simulink model "Houghline_real"  (R2016a)
settings: Solver=VariableStepAuto  StartTime=0.0  StopTime=inf  RelTol=1e-3
undefined symbols (not defined in the file): gray, strel
libraries: visionanalysis x5, visiontransforms x3, visionmorphops x2, visiontextngfix x2, dspvision x1, visionstatistics x1, visionconversions x1
settings Model: Creator=Yewly  LastModifiedBy=Yewly
settings GRTTargetCC: GeneratePreprocessorConditionals=Use local settings

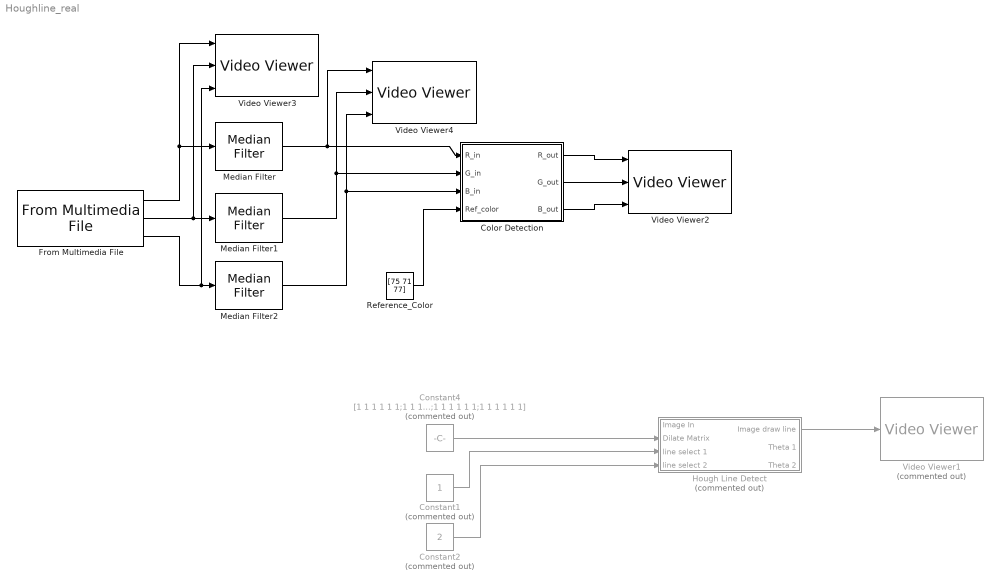
== system Houghline_real ==
  Color Detection : Subsystem
  Constant1 : Constant  Commented=on  OutDataTypeStr=double
  Constant2 : Constant  Commented=on  Value=2  OutDataTypeStr=double
  Constant4 : Constant  Commented=on  Value=[1 1 1 1 1 1;1 1 1 1 1 1;1 1 1 1 1 1;1 1 1 1 1 1;1 1 1 1 1 1;1 1 1 1 1 1]  OutDataTypeStr=boolean
  From Multimedia File : dspvision/From Multimedia File  inputFilename=lane2.mp4  loop=on  numPlays=inf  outputStreams=Video only  videoDataType=single  audioDataType=int16  inheritSampleTime=on  userDefinedSampleTime=1/30  noAudioOutput=off  isIntensityVideo=off  fourcc=RGB  colorVideoFormat=Separate color signals  outputEOF=off  dataOrg=Column-major  audioFrameSize=1024  computeAudioFrameSize=off  outSamplingMode=Sample based
  "Hough Line Detect " : Subsystem  Commented=on
  Median Filter : visionanalysis/Median Filter  nghbood=[11 11]  outSize=Same as input port I  padType=Symmetric  padSrc=Specify via dialog  padVal=0  roundingMode=Floor  overflowMode=off
  Median Filter1 : visionanalysis/Median Filter  nghbood=[11 11]  outSize=Same as input port I  padType=Symmetric  padSrc=Specify via dialog  padVal=0  roundingMode=Floor  overflowMode=off
  Median Filter2 : visionanalysis/Median Filter  nghbood=[11 11]  outSize=Same as input port I  padType=Symmetric  padSrc=Specify via dialog  padVal=0  roundingMode=Floor  overflowMode=off
  Reference_Color : Constant  Value=[75 71 77]  OutDataTypeStr=uint8
  Video Viewer1 : VideoViewer  Commented=on  colormapValue=gray(256)  FigPos=[596.2 615.6 714.4 445.6]
  Video Viewer2 : VideoViewer  imagePorts=separate color signals  colormapValue=gray(256)  FigPos=[459.4 708.4 714.4 445.6]
  Video Viewer3 : VideoViewer  imagePorts=separate color signals  colormapValue=gray(256)  FigPos=[752.2 654.8 714.4 445.6]
  Video Viewer4 : VideoViewer  imagePorts=separate color signals  colormapValue=gray(256)  FigPos=[113.8 832.4 714.4 445.6]
  wires:
  Constant4/1 -> "Hough Line Detect "/2("Dilate Matrix ")
  "Hough Line Detect "/1("Image draw line ") -> Video Viewer1/1
  Constant1/1 -> "Hough Line Detect "/3(line select 1)
  Constant2/1 -> "Hough Line Detect "/4(line select 2)
  From Multimedia File/1 -> Video Viewer3/1, Median Filter/1
  From Multimedia File/2 -> Video Viewer3/2, Median Filter1/1
  From Multimedia File/3 -> Video Viewer3/3, Median Filter2/1
  Median Filter/1 -> Color Detection/1(R_in), Video Viewer4/1
  Median Filter1/1 -> Color Detection/2(G_in), Video Viewer4/2
  Median Filter2/1 -> Color Detection/3(B_in), Video Viewer4/3
  Reference_Color/1 -> Color Detection/4(Ref_color)
  Color Detection/1(R_out) -> Video Viewer2/1
  Color Detection/2(G_out) -> Video Viewer2/2
  Color Detection/3(B_out) -> Video Viewer2/3

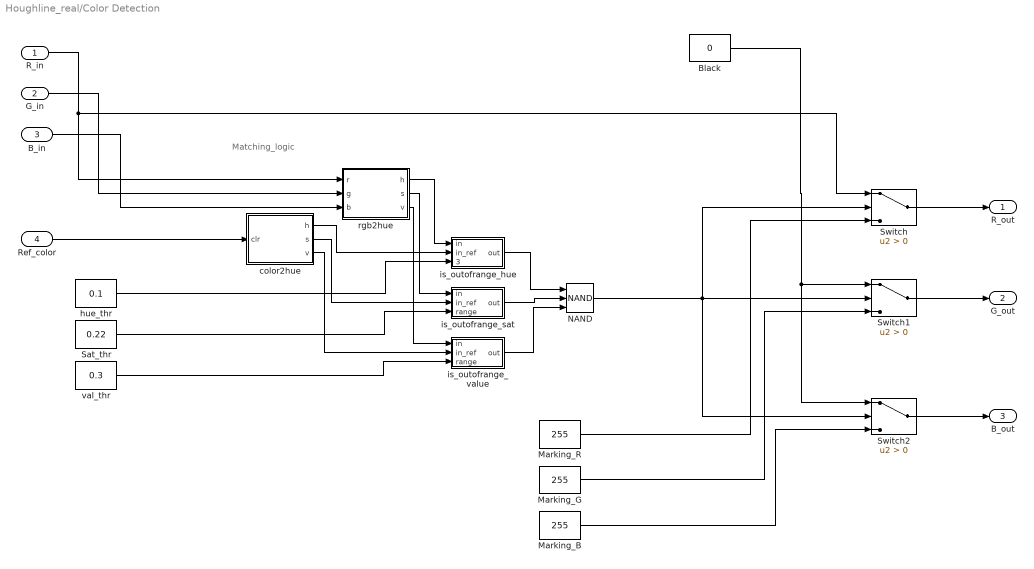
== system Houghline_real/Color Detection ==
  note: Matching_logic
  R_in : Inport
  G_in : Inport  Port=2
  B_in : Inport  Port=3
  Ref_color : Inport  Port=4
  "Black " : Constant  Value=0
  Marking_B : Constant  Value=255
  Marking_G : Constant  Value=255
  Marking_R : Constant  Value=255
  NAND : Logic  Operator=NAND  Inputs=3  IconShape=distinctive  AllPortsSameDT=off  OutDataTypeStr=boolean
  Sat_thr : Constant  Value=0.22
  Switch : Switch  Criteria=u2 > Threshold  OutDataTypeStr=uint8
  Switch1 : Switch  Criteria=u2 > Threshold  OutDataTypeStr=uint8
  Switch2 : Switch  Criteria=u2 > Threshold  OutDataTypeStr=uint8
  color2hue : MATLAB Function  TreatAsAtomicUnit=on
  hue_thr : Constant  Value=0.1
  is_outofrange_hue : Subsystem
  "is_outofrange_sat " : Subsystem
  is_outofrange_value : Subsystem
  rgb2hue : MATLAB Function  TreatAsAtomicUnit=on
  val_thr : Constant  Value=0.3
  R_out : Outport
  G_out : Outport  Port=2
  B_out : Outport  Port=3
  wires:
  NAND/1 -> Switch2/2, Switch1/2, Switch/2
  hue_thr/1 -> is_outofrange_hue/3("threshold ")
  is_outofrange_value/1(out) -> NAND/3
  is_outofrange_hue/1(out) -> NAND/1
  Sat_thr/1 -> "is_outofrange_sat "/3("range ")
  val_thr/1 -> is_outofrange_value/3("range ")
  rgb2hue/3(v) -> is_outofrange_value/1(in)
  color2hue/3(v) -> is_outofrange_value/2(in_ref)
  color2hue/1(h) -> is_outofrange_hue/2(in_ref)
  rgb2hue/1(h) -> is_outofrange_hue/1(in)
  Ref_color/1 -> color2hue/1(clr)
  "is_outofrange_sat "/1(out) -> NAND/2
  color2hue/2(s) -> "is_outofrange_sat "/2(in_ref)
  G_in/1 -> rgb2hue/2(g)
  rgb2hue/2(s) -> "is_outofrange_sat "/1(in)
  B_in/1 -> rgb2hue/3(b)
  R_in/1 -> Switch/1, rgb2hue/1(r)
  Marking_R/1 -> Switch/3
  Switch/1 -> R_out/1
  Switch1/1 -> G_out/1
  Switch2/1 -> B_out/1
  Marking_G/1 -> Switch1/3
  Marking_B/1 -> Switch2/3
  "Black "/1 -> Switch2/1, Switch1/1

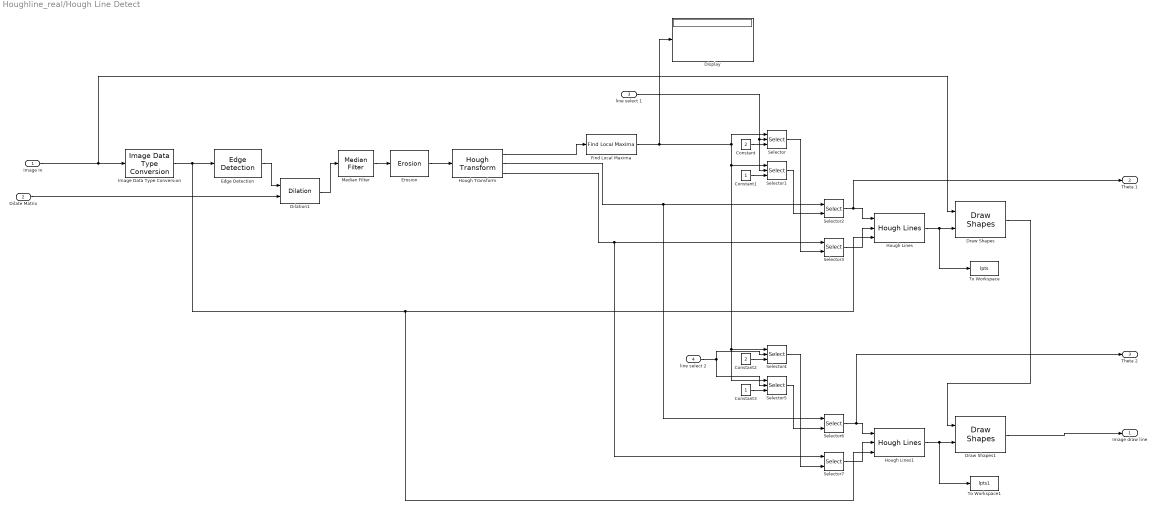
== system Houghline_real/Hough Line Detect  ==
  Image In : Inport
  "Dilate Matrix " : Inport  Port=2
  line select 1 : Inport  Port=3
  line select 2 : Inport  Port=4
  Constant : Constant  Value=2
  Constant1 : Constant
  Constant2 : Constant  Value=2
  Constant3 : Constant
  Dilation1 : visionmorphops/Dilation  nhoodsrc=Input port  strel=[1 1 1 1 1 1;1 1 1 1 1 1;1 1 1 1 1 1;1 1 1 1 1 1;1 1 1 1 1 1;1 1 1 1 1 1]
  Display : Display
  Draw Shapes : visiontextngfix/Draw Shapes  shape=Lines  fill=off  lineWidth=10  fillClrSource=Specify via dialog  display=White  intensity=200  color=255  opacity=0.6  viewport=Entire image  antialiasing=off  inType=Obsolete  imagePorts=One multidimensional signal  prodOutputMode=Binary point scaling  prodOutputWordLength=32  prodOutputFracLength=14  memoryMode=Specify word length  memoryWordLength=16  memoryFracLength=14  roundingMode=Floor  overflowMode=off
  Draw Shapes1 : visiontextngfix/Draw Shapes  shape=Lines  fill=off  lineWidth=10  fillClrSource=Specify via dialog  display=White  intensity=200  color=255  opacity=0.6  viewport=Entire image  antialiasing=off  inType=Obsolete  imagePorts=One multidimensional signal  prodOutputMode=Binary point scaling  prodOutputWordLength=32  prodOutputFracLength=14  memoryMode=Specify word length  memoryWordLength=16  memoryFracLength=14  roundingMode=Floor  overflowMode=off
  Edge Detection : visionanalysis/Edge Detection  method=Sobel  outputType=Binary image  userDefinedThreshold=off  thresholdSource=Input port  threshold=20  thresholdTuning=4  edgeThinning=on  threshold_canny=[0.25 0.60]  autoPercent=70  sigma=1  prodOutputMode=Binary point scaling  prodOutputWordLength=32  prodOutputFracLength=8  roundingMode=Floor  overflowMode=off
  Erosion : visionmorphops/Erosion  nhoodsrc=Specify via dialog  strel=strel('square',12)
  Find Local Maxima : visionstatistics/Find Local Maxima  num_peaks=5  nhood_size=[5 7]  src_thresh=Obsolete9b  src_thresh_inuse=Specify via dialog  threshold=10  inputIsHough=on  dt_peak=uint32  isOutVarDim=on  dt_count=uint32
  Hough Lines : visiontransforms/Hough Lines  sineCompMethod=Trigonometric function  thetaRes=pi/180  firstCoeffMode=Specify word length  firstCoeffWordLength=16  firstCoeffFracLength=15  prodOutputMode=Binary point scaling  prodOutputWordLength=32  prodOutputFracLength=16  roundingMode=Nearest  overflowMode=on
  Hough Lines1 : visiontransforms/Hough Lines  sineCompMethod=Trigonometric function  thetaRes=pi/180  firstCoeffMode=Specify word length  firstCoeffWordLength=16  firstCoeffFracLength=15  prodOutputMode=Binary point scaling  prodOutputWordLength=32  prodOutputFracLength=16  roundingMode=Nearest  overflowMode=on
  Hough Transform : visiontransforms/Hough Transform  theta_res=pi/360  rho_res=1  out_theta_rho=on  outdtmode=double  firstCoeffMode=Binary point scaling  firstCoeffWordLength=16  firstCoeffFracLength=14  secondCoeffMode=Binary point scaling  secondCoeffWordLength=32  secondCoeffFracLength=16  outputMode=Binary point scaling  outputWordLength=16  outputFracLength=0  accumMode=Binary point scaling  accumWordLength=32  accumFracLength=20  prodOutputMode=Binary point scaling  prodOutputWordLength=32  prodOutputFracLength=20  memoryMode=Binary point scaling  memoryWordLength=32  memoryFracLength=16  roundingMode=Nearest  overflowMode=on
  Image Data Type Conversion : visionconversions/Image Data Type Conversion  outDT=double  isSigned=on  wordLen=16  numFracBits=0
  Median Filter : visionanalysis/Median Filter  nghbood=[3 3]  outSize=Same as input port I  padType=Symmetric  padSrc=Specify via dialog  padVal=0  roundingMode=Floor  overflowMode=off
  Selector : Selector  NumberOfDimensions=2  InputPortWidth=2  IndexOptions=Index vector (port),Index vector (port)  Indices=1,1  OutputSizes=1,1
  Selector1 : Selector  NumberOfDimensions=2  InputPortWidth=2  IndexOptions=Starting index (port),Index vector (port)  Indices=1,1  OutputSizes=1,1
  Selector{2..3,6..7} (4 alike) : Selector  NumberOfDimensions=2  InputPortWidth=3  IndexOptions=Select all,Index vector (port)  Indices=[1 3],1  OutputSizes=1,1
  Selector4 : Selector  NumberOfDimensions=2  InputPortWidth=2  IndexOptions=Index vector (port),Index vector (port)  Indices=2,1  OutputSizes=1,1
  Selector5 : Selector  NumberOfDimensions=2  InputPortWidth=2  IndexOptions=Index vector (port),Index vector (port)  Indices=2,1  OutputSizes=1,1
  To Workspace : ToWorkspace  VariableName=lpts  SampleTime=-1
  To Workspace1 : ToWorkspace  VariableName=lpts1  SampleTime=-1
  "Image draw line " : Outport
  Theta 1 : Outport  Port=2
  Theta 2 : Outport  Port=3
  wires:
  Selector5/1 -> Selector6/2
  Draw Shapes1/1 -> "Image draw line "/1
  Constant1/1 -> Selector1/3
  Constant3/1 -> Selector5/3
  Selector3/1 -> Hough Lines/2
  Hough Transform/3 -> Selector7/1, Selector3/1
  Selector4/1 -> Selector7/2
  Hough Lines/1 -> To Workspace/1, Draw Shapes/2
  Hough Transform/1 -> Find Local Maxima/1
  Edge Detection/1 -> Dilation1/1
  Selector7/1 -> Hough Lines1/2
  Hough Lines1/1 -> To Workspace1/1, Draw Shapes1/2
  Selector1/1 -> Selector2/2
  Constant2/1 -> Selector4/3
  Image In/1 -> Image Data Type Conversion/1, Draw Shapes/1
  Hough Transform/2 -> Selector6/1, Selector2/1
  Dilation1/1 -> Median Filter/1
  Selector/1 -> Selector3/2
  Erosion/1 -> Hough Transform/1
  Draw Shapes/1 -> Draw Shapes1/1
  Median Filter/1 -> Erosion/1
  "Dilate Matrix "/1 -> Dilation1/2
  Selector2/1 -> Theta 1/1, Hough Lines/1
  Selector6/1 -> Theta 2/1, Hough Lines1/1
  line select 1/1 -> Selector1/2, Selector/2
  Constant/1 -> Selector/3
  line select 2/1 -> Selector5/2, Selector4/2
  Image Data Type Conversion/1 -> Hough Lines1/3, Hough Lines/3, Edge Detection/1
  Find Local Maxima/1 -> Display/1, Selector5/1, Selector4/1, Selector1/1, Selector/1

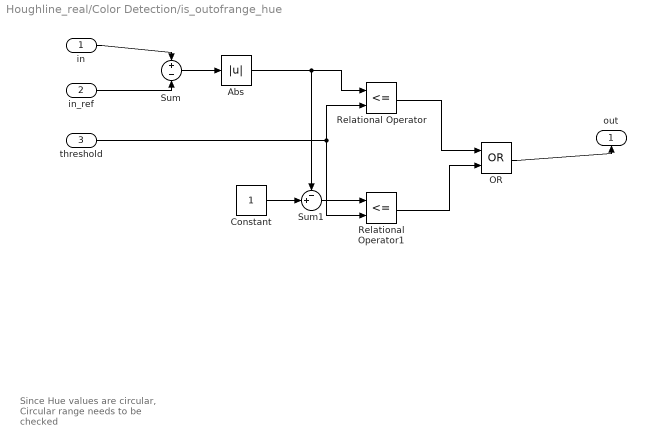
== system Houghline_real/Color Detection/is_outofrange_hue ==
  note: Since Hue values are circular, Circular range needs to be checked
  in : Inport
  in_ref : Inport  Port=2
  "threshold " : Inport  Port=3
  Abs : Abs
  Constant : Constant
  "OR " : Logic  Operator=OR  AllPortsSameDT=off  OutDataTypeStr=boolean
  Relational Operator : RelationalOperator  Operator=<=  OutDataTypeStr=boolean
  Relational Operator1 : RelationalOperator  Operator=<=  OutDataTypeStr=boolean
  Sum : Sum  Inputs=+|-
  Sum1 : Sum  Inputs=-+|
  out : Outport
  wires:
  in/1 -> Sum/1
  in_ref/1 -> Sum/2
  Sum/1 -> Abs/1
  Abs/1 -> Sum1/1, Relational Operator/1
  "threshold "/1 -> Relational Operator1/2, Relational Operator/2
  Constant/1 -> Sum1/2
  Sum1/1 -> Relational Operator1/1
  Relational Operator/1 -> "OR "/1
  Relational Operator1/1 -> "OR "/2
  "OR "/1 -> out/1

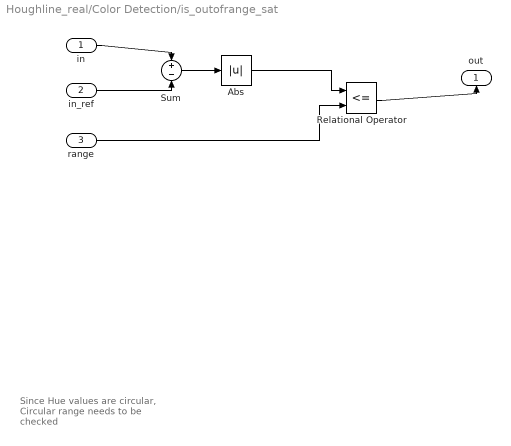
== system Houghline_real/Color Detection/is_outofrange_sat  ==
  note: Since Hue values are circular, Circular range needs to be checked
  in : Inport
  in_ref : Inport  Port=2
  "range " : Inport  Port=3
  Abs : Abs
  Relational Operator : RelationalOperator  Operator=<=  OutDataTypeStr=boolean
  Sum : Sum  Inputs=+|-
  out : Outport
  wires:
  in/1 -> Sum/1
  in_ref/1 -> Sum/2
  Sum/1 -> Abs/1
  Abs/1 -> Relational Operator/1
  "range "/1 -> Relational Operator/2
  Relational Operator/1 -> out/1

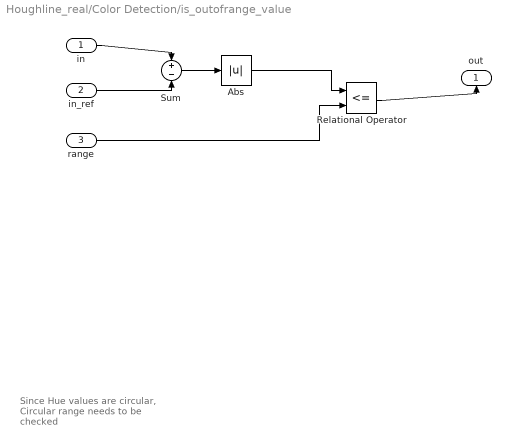
== system Houghline_real/Color Detection/is_outofrange_value ==
  note: Since Hue values are circular, Circular range needs to be checked
  in : Inport
  in_ref : Inport  Port=2
  "range " : Inport  Port=3
  Abs : Abs
  Relational Operator : RelationalOperator  Operator=<=  OutDataTypeStr=boolean
  Sum : Sum  Inputs=+|-
  out : Outport
  wires:
  in/1 -> Sum/1
  in_ref/1 -> Sum/2
  Sum/1 -> Abs/1
  Abs/1 -> Relational Operator/1
  "range "/1 -> Relational Operator/2
  Relational Operator/1 -> out/1

== matlab function Houghline_real/Color Detection/rgb2hue ==
  data: r input; h output; g input; b input; s output; v output
function [h,s,v] = rgb2hue(r,g,b)
%#codegen

sz = size(r);
r_re = double(reshape(r,[sz(1)*sz(2),1]))/255.0;
g_re = double(reshape(g,[sz(1)*sz(2),1]))/255.0;
b_re = double(reshape(b,[sz(1)*sz(2),1]))/255.0;
hsv = rgb2hsv([r_re,g_re,b_re]);
h = reshape(hsv(:,1), sz);
s = reshape(hsv(:,2), sz);
v = reshape(hsv(:,3), sz);

== matlab function Houghline_real/Color Detection/color2hue ==
  data: clr input; h output; s output; v output
function [h,s,v] = color2hue(clr)
%#codegen

hsv = rgb2hsv(double(clr')/255.0);
h = hsv(1);
s = hsv(2);
v = hsv(3);
